simulink model "testModel"  (R2016b)
settings: Solver=FixedStepAuto  StartTime=0.0  StopTime=20  FixedStep=1e-3  RelTol=1e-3
values from neighbouring files (symbols this model uses):
  Jtarget = 2.345e-4    (= 0.0002345)    [testEstimation.m]
libraries: simulink x2
settings Model: Creator=jelavice  LastModifiedBy=jelavice

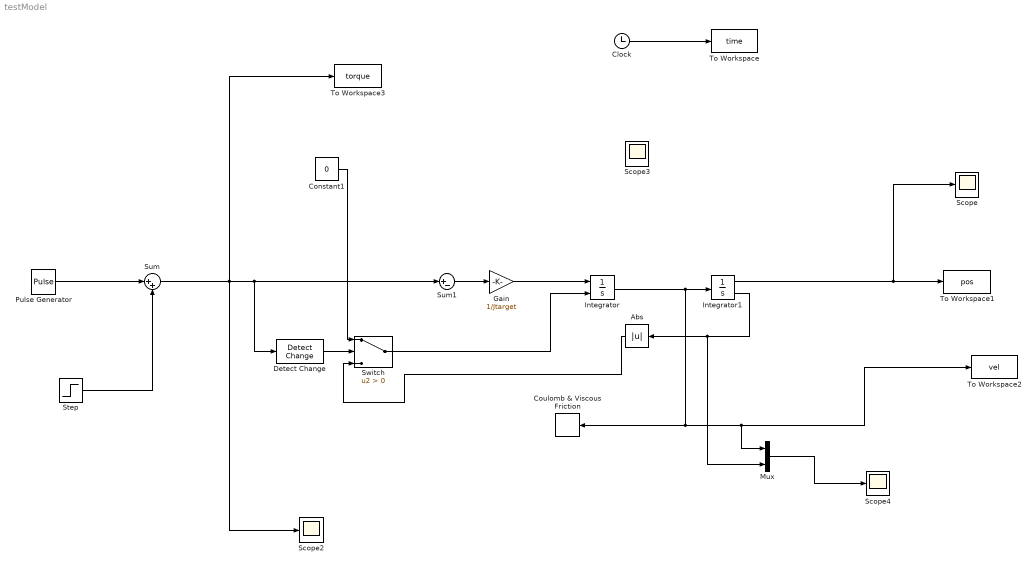
== system testModel ==
  Abs : Abs
  Clock : Clock
  Constant1 : Constant  Value=0
  Coulomb & Viscous Friction : simulink/Discontinuities/Coulomb & Viscous Friction  offset=3  gain=0
  Detect Change : simulink/Logic and Bit Operations/Detect Change  vinit=0  OutDataTypeStr=boolean
  Gain : Gain  Gain=1/Jtarget
  Integrator : Integrator  ExternalReset=level hold
  Integrator1 : Integrator  LimitOutput=on  UpperSaturationLimit=pi/2  LowerSaturationLimit=-pi/2  ShowSaturationPort=on
  Mux : Mux  Inputs=2
  Pulse Generator : DiscretePulseGenerator  PulseType=Time based  Amplitude=10  Period=4  PulseWidth=50  PhaseDelay=2
  Scope{,2..4} (4 alike) : Scope
  Step : Step  Time=2  After=-5  SampleTime=0
  Sum : Sum  Inputs=|++
  Sum1 : Sum  Inputs=|+-
  Switch : Switch  Criteria=u2 > Threshold
  To Workspace : ToWorkspace  VariableName=time  SampleTime=-1
  To Workspace1 : ToWorkspace  VariableName=pos  SampleTime=-1
  To Workspace2 : ToWorkspace  VariableName=vel  SampleTime=-1
  To Workspace3 : ToWorkspace  VariableName=torque  SampleTime=-1
  wires:
  Integrator/1 -> Integrator1/1, Coulomb & Viscous Friction/1, Mux/1, To Workspace2/1
  Clock/1 -> To Workspace/1
  Integrator1/1 -> Scope/1, To Workspace1/1
  Gain/1 -> Integrator/1
  Pulse Generator/1 -> Sum/1
  Step/1 -> Sum/2
  Integrator1/2 -> Mux/2, Abs/1
  Sum1/1 -> Gain/1
  Abs/1 -> Switch/3
  Switch/1 -> Integrator/2
  Constant1/1 -> Switch/1
  Detect Change/1 -> Switch/2
  Mux/1 -> Scope4/1
  Sum/1 -> Detect Change/1, Sum1/1, Scope2/1, To Workspace3/1
